simulink model "amortiguacion"  (R2023b)
settings: Solver=ode45  StartTime=0  StopTime=20  FixedStep=1  RelTol=1e-3
undefined symbols (not defined in the file): cc, kc, kr, mc, mr, mu
settings Model: Creator=anruk  LastModifiedBy=anruk

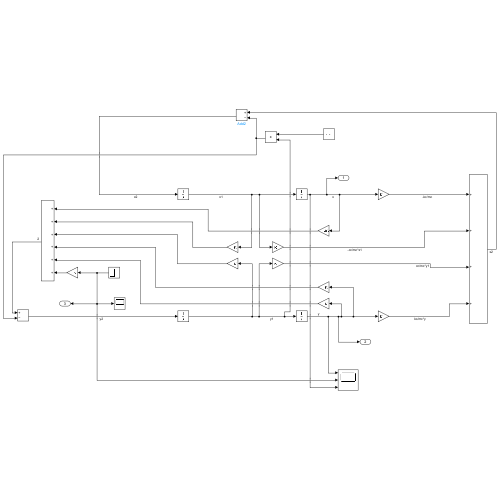
[thumbnail: Simulink's stored preview of the top-level diagram]
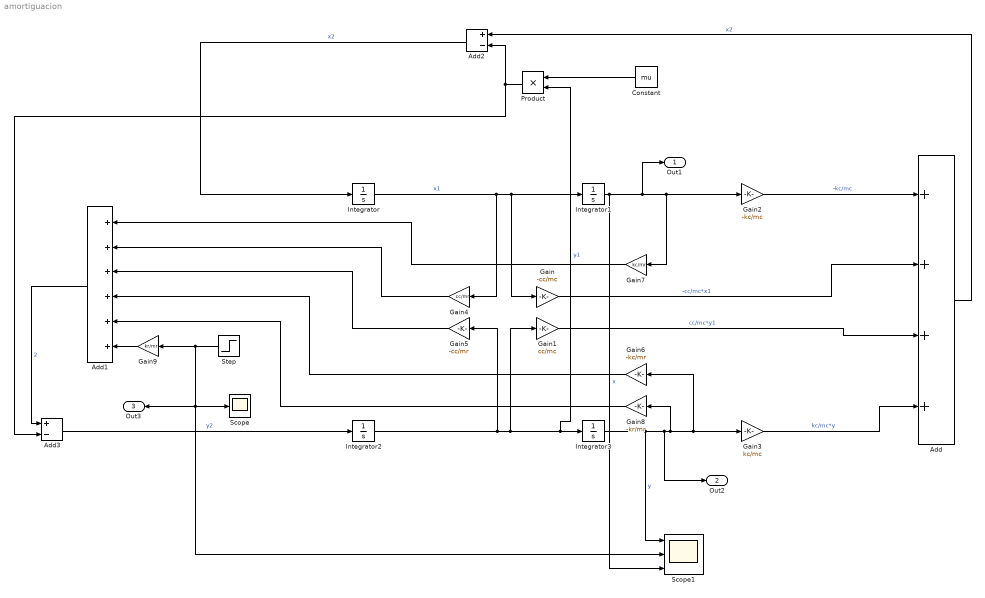
== system amortiguacion ==
  Add : Sum  Inputs=++++
  Add1 : Sum  Inputs=++++++
  Add2 : Sum  Inputs=+-
  Add3 : Sum  Inputs=+-
  Constant : Constant  Value=mu
  Gain : Gain  Gain=-cc/mc
  Gain1 : Gain  Gain=cc/mc
  Gain2 : Gain  Gain=-kc/mc
  Gain3 : Gain  Gain=kc/mc
  Gain4 : Gain  Gain=cc/mr
  Gain5 : Gain  Gain=-cc/mr
  Gain6 : Gain  Gain=-kc/mr
  Gain7 : Gain  Gain=kc/mr
  Gain8 : Gain  Gain=-kr/mr
  Gain9 : Gain  Gain=kr/mr
  Integrator{,1..3} (4 alike) : Integrator
  Product : Product
  Scope : Scope
  Scope1 : Scope  NumInputPorts=3
  Step : Step  SampleTime=0
  Out1 : Outport
  Out2 : Outport  Port=2
  Out3 : Outport  Port=3
  wires:
  Integrator/1 -> Gain4/1, Gain/1, Integrator1/1  "x1"
  Integrator2/1 -> Product/2, Integrator3/1, Gain1/1, Gain5/1  "y1"
  Integrator3/1 -> Scope1/1, Out2/1, Gain8/1, Gain6/1, Gain3/1  "y"
  Integrator1/1 -> Scope1/3, Out1/1, Gain7/1, Gain2/1  "x"
  Gain/1 -> Add/2  "-cc/mc*x1"
  Gain1/1 -> Add/3  "cc/mc*y1"
  Gain3/1 -> Add/4  "kc/mc*y"
  Gain2/1 -> Add/1  "-kc/mc"
  Gain5/1 -> Add1/3
  Gain4/1 -> Add1/2
  Gain6/1 -> Add1/4
  Gain7/1 -> Add1/1
  Gain8/1 -> Add1/5
  Gain9/1 -> Add1/6
  Step/1 -> Scope/1, Out3/1, Scope1/2, Gain9/1
  Add/1 -> Add2/1  "x2"
  Add2/1 -> Integrator/1  "x2"
  Constant/1 -> Product/1
  Product/1 -> Add3/2, Add2/2
  Add3/1 -> Integrator2/1  "y2"
  Add1/1 -> Add3/1  "2"
